simulink model "system_model"  (R2025b)
settings: Solver=ode4  StartTime=0.0  StopTime=T_sim  FixedStep=1e-6  MaxStep=6e-5  RelTol=1e-6
values from neighbouring files (symbols this model uses):
  params = Simulink.Parameter(params_data)    [calc_simulation_params.m]
undefined symbols (not defined in the file or in its folder): p0, Ts
settings Model: Creator=kevin  LastModifiedBy=kevin
settings DataIOCC: TimeSaveName=t_out

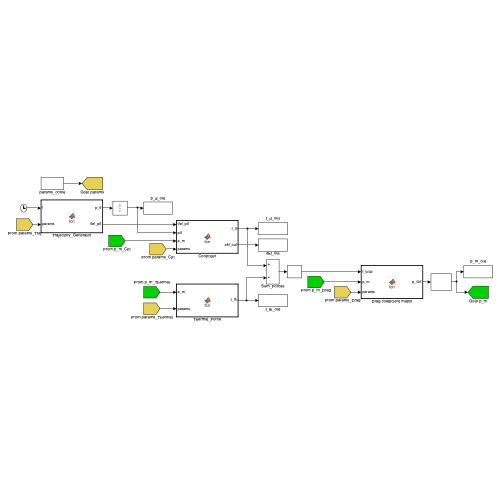
[thumbnail: Simulink's stored preview of the top-level diagram]
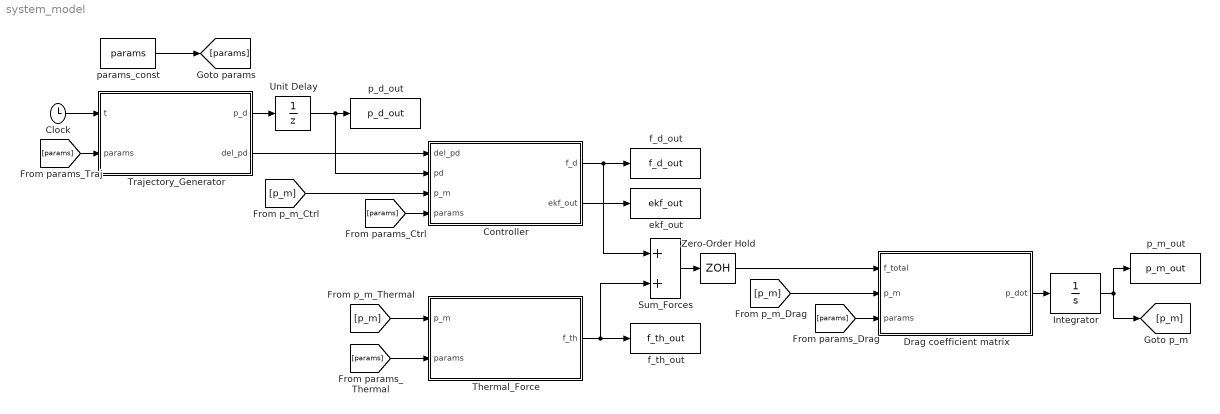
== system system_model ==
  Clock : Clock
  Controller : MATLAB Function  TreatAsAtomicUnit=on
  Drag coefficient matrix : MATLAB Function  TreatAsAtomicUnit=on
  Integrator : Integrator  InitialCondition=p0
  Sum_Forces : Sum
  Thermal_Force : MATLAB Function  TreatAsAtomicUnit=on
  Trajectory_Generator : MATLAB Function  TreatAsAtomicUnit=on
  Unit Delay : UnitDelay  InitialCondition=p0  SampleTime=Ts  HasFrameUpgradeWarning=on
  Zero-Order Hold : ZeroOrderHold  SampleTime=Ts
  ekf_out : ToWorkspace  VariableName=ekf_out  SampleTime=Ts
      settings: Save2DSignal=2-D array (concatenate along first dimension)
  f_d_out : ToWorkspace  VariableName=f_d_out  SampleTime=Ts
      settings: Save2DSignal=2-D array (concatenate along first dimension)
  f_th_out : ToWorkspace  VariableName=f_th_out  SampleTime=Ts
      settings: Save2DSignal=2-D array (concatenate along first dimension)
  p_d_out : ToWorkspace  VariableName=p_d_out  SampleTime=Ts
      settings: Save2DSignal=2-D array (concatenate along first dimension)
  p_m_out : ToWorkspace  VariableName=p_m_out  SampleTime=-1
      settings: Save2DSignal=2-D array (concatenate along first dimension)
  params_const : Constant  Value=params  OutDataTypeStr=Bus: ParamsBus
  wires:
  Clock/1 -> Trajectory_Generator/1(t)
  params_const/1 -> [params]
  [params] -> Drag coefficient matrix/3(params)
  [params] -> Trajectory_Generator/2(params)
  Trajectory_Generator/1(p_d) -> Unit Delay/1
  [p_m] -> Thermal_Force/1(p_m)
  [params] -> Thermal_Force/2(params)
  Thermal_Force/1(f_th) -> Sum_Forces/2, f_th_out/1
  Sum_Forces/1 -> Zero-Order Hold/1
  [p_m] -> Drag coefficient matrix/2(p_m)
  Zero-Order Hold/1 -> Drag coefficient matrix/1(f_total)
  Drag coefficient matrix/1(p_dot) -> Integrator/1
  Integrator/1 -> [p_m], p_m_out/1
  Unit Delay/1 -> Controller/2(pd), p_d_out/1
  Trajectory_Generator/2(del_pd) -> Controller/1(del_pd)
  [params] -> Controller/4(params)
  Controller/2(ekf_out) -> ekf_out/1
  Controller/1(f_d) -> Sum_Forces/1, f_d_out/1
  [p_m] -> Controller/3(p_m)

== matlab function system_model/Controller ==
  settings: updateMethod=DISCRETE  sampleTime=Ts
  data: del_pd input size=3; pd input; f_d output size=3; p_m input size=3; params input; ekf_out output size=4
function [f_d, ekf_out] = fcn(del_pd, pd, p_m, params)
%#codegen
    [f_d, ekf_out] = motion_control_law(del_pd, pd, p_m, params);
end

== matlab function system_model/Trajectory_Generator ==
  settings: updateMethod=DISCRETE  sampleTime=Ts
  data: t input; p_d output size=3; params input; del_pd output
function [p_d, del_pd] = fcn(t, params)
%#codegen
    [p_d, del_pd] = trajectory_generator(t, params);
end

== matlab function system_model/Thermal_Force ==
  settings: updateMethod=DISCRETE  sampleTime=Ts
  data: p_m input size=3; f_th output size=3; params input
function f_th = fcn(p_m, params)
%#codegen
    if params.thermal.enable > 0.5
        f_th = calc_thermal_force(p_m, params);
    else
        f_th = zeros(3, 1);
    end
end

== matlab function system_model/Drag coefficient matrix ==
  settings: updateMethod=CONTINUOUS
  data: f_total input size=3; p_dot output size=3; p_m input size=3; params input
function p_dot = fcn(f_total, p_m, params)
%#codegen
    [Gamma_inv, ~] = calc_gamma_inv(p_m, params);
    p_dot = Gamma_inv * f_total;
end
